simulink model "sl_puma_hw7"  (R2014b)
settings: Solver=ode45  StartTime=0.0  StopTime=time(end-1)  FixedStep=.001  RelTol=1e-3
InitFcn:
  | problem_1
values from neighbouring files (symbols this model uses):
  p560 = p560.nofriction    [problem_1.m]
undefined symbols (not defined in the file or in its folder): P
libraries: roblocks x2
settings Model: ExtModeTrigMode=oneshot  ExtModeArmWhenConnect=off  Creator=pic  LastModifiedBy=root
settings DataIOCC: LimitDataPoints=off  SignalLoggingSaveFormat=ModelDataLogs  SignalLogging=off  ReturnWorkspaceOutputs=on
settings OptimizationCC: BlockReduction=off  BooleanDataType=off  UseDivisionForNetSlopeComputation=off  ExpressionDepthLimit=2147483647  InitFltsAndDblsToZero=on  SimCompilerOptimization=off
settings DebuggingCC: SaveWithParameterizedLinksMsg=none  UnderspecifiedInitializationDetection=Classic  MergeDetectMultiDrivingBlocksExec=none  SignalResolutionControl=TryResolveAllWithWarning  SolverPrmCheckMsg=none  MultiTaskDSMMsg=warning  MultiTaskCondExecSysMsg=none  FcnCallInpInsideContextMsg=EnableAllAsWarning  FrameProcessingCompatibilityMsg=error  StateNameClashWarn=warning
settings HardwareCC: TargetUnknown=on
settings RTWCC: RTWCompilerOptimization=off
settings GRTTargetCC: ModelReferenceCompliant=off  ParMdlRefBuildCompliant=off  CompOptLevelCompliant=off  CombineOutputUpdateFcns=off  MatFileLogging=off  GRTInterface=on

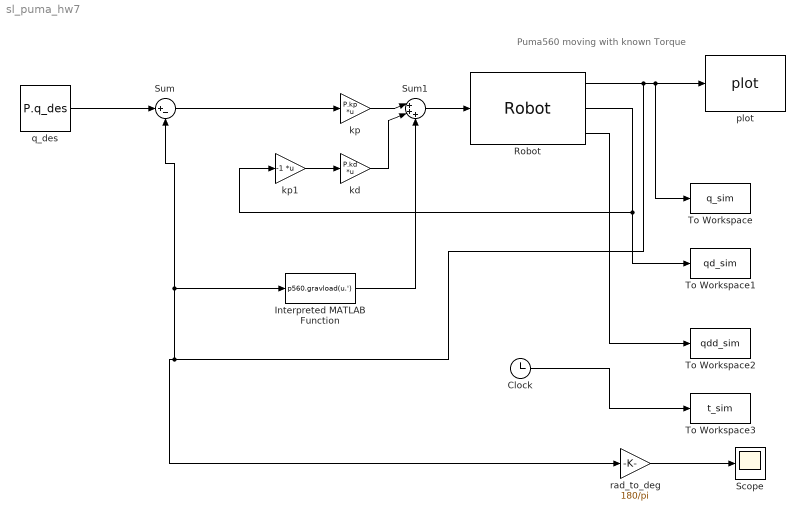
== system sl_puma_hw7 ==
  note: Puma560 moving with known Torque
  Clock : Clock
  Interpreted MATLAB Function : MATLABFcn  MATLABFcn=p560.gravload(u.')
  Robot : roblocks/Dynamics/Robot  robot=p560.nofriction  q0=[0 0 0 0 0 0]
  Scope : Scope
      settings: YMin=-80  YMax=80  SaveName=ScopeData2
  Sum : Sum  Inputs=|+-
  Sum1 : Sum  Inputs=|+++
  To Workspace : ToWorkspace  VariableName=q_sim  SampleTime=-1
  To Workspace1 : ToWorkspace  VariableName=qd_sim  SampleTime=-1
  To Workspace2 : ToWorkspace  VariableName=qdd_sim  SampleTime=-1
  To Workspace3 : ToWorkspace  VariableName=t_sim  SampleTime=-1
  kd : Gain  Gain=P.kd  Multiplication=Matrix(K*u)
  kp : Gain  Gain=P.kp  Multiplication=Matrix(K*u)
  kp1 : Gain  Gain=-1  Multiplication=Matrix(K*u)
  plot : roblocks/Robot Graphics/plot  robot=p560  fps=25  holdplot=on
  q_des : Constant  Value=P.q_des
  rad_to_deg : Gain  Gain=180/pi
  wires:
  Robot/1 -> rad_to_deg/1, Sum/2, Interpreted MATLAB Function/1, To Workspace/1, plot/1
  Robot/3 -> To Workspace2/1
  Robot/2 -> kp1/1, To Workspace1/1
  q_des/1 -> Sum/1
  Sum/1 -> kp/1
  Clock/1 -> To Workspace3/1
  kp/1 -> Sum1/1
  Sum1/1 -> Robot/1
  rad_to_deg/1 -> Scope/1
  Interpreted MATLAB Function/1 -> Sum1/3
  kd/1 -> Sum1/2
  kp1/1 -> kd/1
